simulink model "sampling_3_phases"  (R2021a)
settings: Solver=VariableStepAuto  StartTime=0.0  StopTime=0.01  RelTol=1e-3
settings Model: Creator=Mrittik  LastModifiedBy=Mrittik

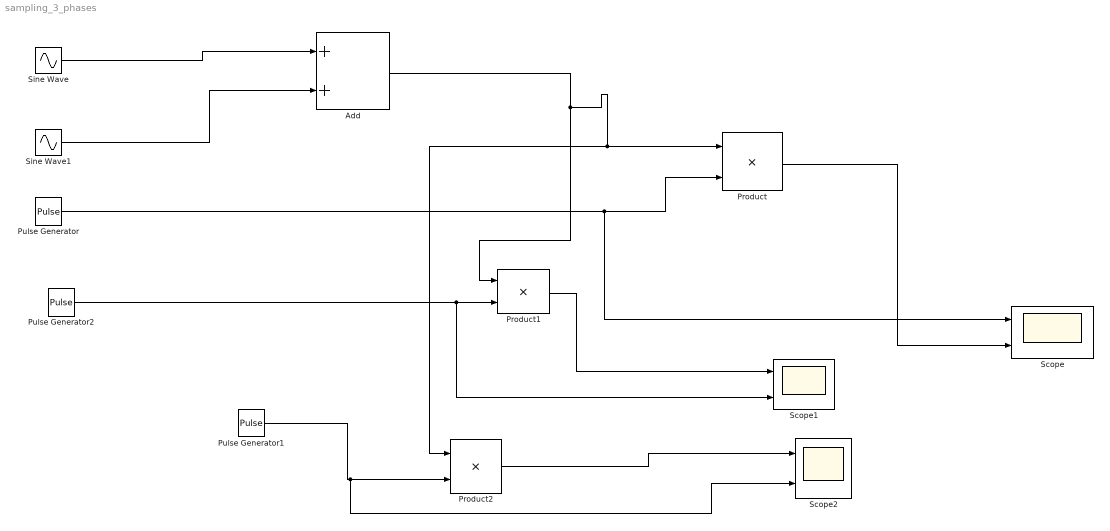
== system sampling_3_phases ==
  Add : Sum
  Product : Product
  Product1 : Product
  Product2 : Product
  Pulse Generator : DiscretePulseGenerator  PulseType=Time based  Period=1/2000  PulseWidth=50
  Pulse Generator1 : DiscretePulseGenerator  PulseType=Time based  Period=1/1000  PulseWidth=50
  Pulse Generator2 : DiscretePulseGenerator  PulseType=Time based  Period=1/3000  PulseWidth=50
  Scope : Scope  NumInputPorts=2
  Scope1 : Scope  NumInputPorts=2
  Scope2 : Scope  NumInputPorts=2
  Sine Wave : Sin  Frequency=1000  SampleTime=0
  Sine Wave1 : Sin  Frequency=1000  SampleTime=0
  wires:
  Sine Wave/1 -> Add/1
  Sine Wave1/1 -> Add/2
  Add/1 -> Product1/1, Product2/1, Product/1
  Product/1 -> Scope/2
  Pulse Generator/1 -> Scope/1, Product/2
  Pulse Generator2/1 -> Scope1/2, Product1/2
  Pulse Generator1/1 -> Scope2/2, Product2/2
  Product1/1 -> Scope1/1
  Product2/1 -> Scope2/1
